simulink model "encoderfinal"  (R2021a)
settings: Solver=FixedStepAuto  StartTime=0.0  StopTime=100  RelTol=1e-3  EnableMultiTasking=on
libraries: arduinolib x5
settings Model: SILPILModeSetting=veronly  ExtModeTrigDuration=2  Creator=admin  LastModifiedBy=admin
settings OptimizationCC: EnhancedBackFolding=on  PassReuseOutputArgsAs=Individual arguments  ZeroExternalMemoryAtStartup=off  ZeroInternalMemoryAtStartup=off  MaxStackSize=64  OptimizeBlockOrder=speed  DifferentSizesBufferReuse=on  OptimizationCustomize=off  EfficientTunableParamExpr=on
settings DebuggingCC: ParameterTunabilityLossMsg=error
settings HardwareCC: ProdBitPerPointer=32  ProdBitPerSizeT=32  ProdBitPerPtrDiffT=32  ProdLargestAtomicInteger=Long  ProdLargestAtomicFloat=Double  ProdWordSize=32  ProdHWDeviceType=ARM Compatible->ARM Cortex
settings SFSimCC: MATLABDynamicMemAlloc=off
settings RTWCC: SystemTargetFile=ert.tlc  HardwareBoard=Arduino Due  TemplateMakefile=ert_default_tmf  Toolchain=Arduino ARM  BuildConfiguration=Faster Runs
settings CodeAppCC: ForceParamTrailComments=on  IgnoreCustomStorageClasses=off  OperatorAnnotations=on  SimulinkDataObjDesc=on  SFDataObjDesc=on  InsertBlockDesc=on
settings ERTTargetCC: SupportContinuousTime=on  SupportVariableSizeSignals=on  ExtModeTransport=3  ExtModeStaticAlloc=on  ExtModeStaticAllocSize=24576  ExtModeMexFile=ext_xcp  ExtModeIntrfLevel=Level2 - Open

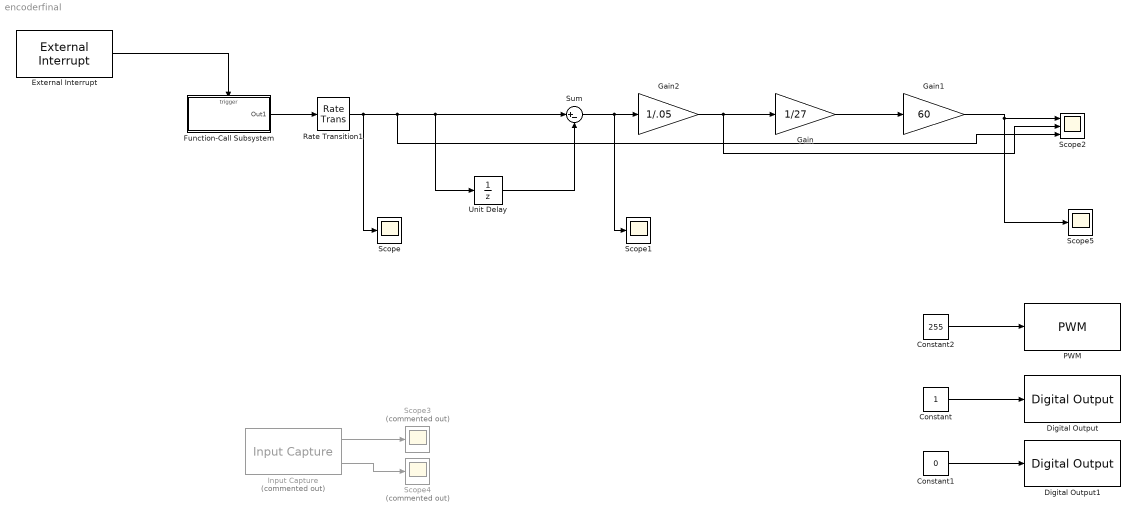
== system encoderfinal ==
  Constant : Constant
  Constant1 : Constant  Value=0
  Constant2 : Constant  Value=255
  Digital Output : arduinolib/Digital Output  pinNumber=5  Direction=output  blockPlatform=arduino
  Digital Output1 : arduinolib/Digital Output  pinNumber=6  Direction=output  blockPlatform=arduino
  External Interrupt : arduinolib/External Interrupt  Pin=2  PullUp=off  Mode=RISING  InterruptSimulationInput=off
      settings: SourceProductBaseCode=ARDUINO
  Function-Call Subsystem : Subsystem  TreatAsAtomicUnit=on
  Gain : Gain  Gain=1/27
  Gain1 : Gain  Gain=60
  Gain2 : Gain  Gain=1/.05
  Input Capture : arduinolib/Input Capture  Commented=on  InputCapturePinNumber=2  SampleTime=0.1
      settings: SourceProductBaseCode=ARDUINO
  PWM : arduinolib/PWM  pinNumber=4  frequencyType=Default  desiredFrequency=490.2  achievableFrequency=490.2
  Rate Transition1 : RateTransition  Deterministic=off
  Scope : Scope
  Scope1 : Scope
  Scope2 : Scope  NumInputPorts=3
  Scope3 : Scope  Commented=on
  Scope4 : Scope  Commented=on
  Scope5 : Scope
  Sum : Sum  Inputs=|+-
  Unit Delay : UnitDelay  SampleTime=.05  HasFrameUpgradeWarning=on
  wires:
  External Interrupt/1 -> Function-Call Subsystem/Trigger
  Function-Call Subsystem/1(Out1) -> Rate Transition1/1
  Rate Transition1/1 -> Scope2/3, Unit Delay/1, Sum/1, Scope/1
  Unit Delay/1 -> Sum/2
  Sum/1 -> Scope1/1, Gain2/1
  Constant/1 -> Digital Output/1
  Constant1/1 -> Digital Output1/1
  Constant2/1 -> PWM/1
  Gain/1 -> Gain1/1
  Gain1/1 -> Scope5/1, Scope2/1
  Input Capture/1 -> Scope3/1
  Input Capture/2 -> Scope4/1
  Gain2/1 -> Scope2/2, Gain/1

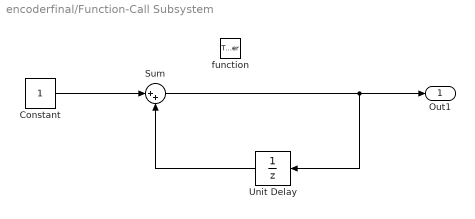
== system encoderfinal/Function-Call Subsystem ==
  function : TriggerPort  TriggerType=function-call  VariantControl=(inherit)
  Constant : Constant  SampleTime=-1
  Sum : Sum  Inputs=|++
  Unit Delay : UnitDelay  SampleTime=-1  HasFrameUpgradeWarning=on
  Out1 : Outport  VectorParamsAs1DForOutWhenUnconnected=off
  wires:
  Unit Delay/1 -> Sum/2
  Constant/1 -> Sum/1
  Sum/1 -> Unit Delay/1, Out1/1
